simulink model "TestCurrentMotor"  (R2013b)
settings: Solver=ode45  StartTime=0.0  StopTime=inf  RelTol=1e-3
libraries: simulink x1
settings Model: Creator=eugenio  LastModifiedBy=eyime
settings DataIOCC: SignalLoggingSaveFormat=ModelDataLogs
settings OptimizationCC: ExpressionDepthLimit=2147483647
settings DebuggingCC: FcnCallInpInsideContextMsg=UseLocalSettings  StateNameClashWarn=warning
settings SFSimCC: SimParseCustomCode=off
settings GRTTargetCC: CombineOutputUpdateFcns=off  GRTInterface=on
settings SimMechanicsCC: VisDuringSimulation=on
settings ConfigurationSet: Description=SimMechanics 2G

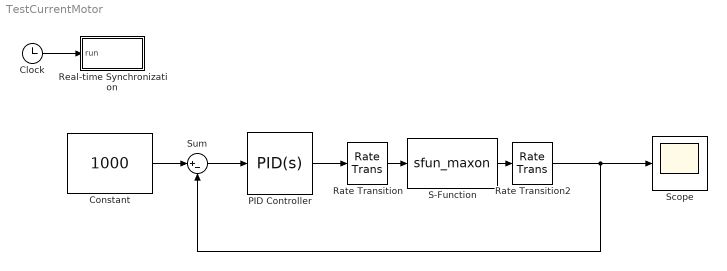
== system TestCurrentMotor ==
  Clock : Clock
  Constant : Constant  Value=1000
  PID Controller : simulink/Continuous/PID Controller  Controller=PID  TimeDomain=Continuous-time  SampleTime=1  IntegratorMethod=Forward Euler  FilterMethod=Forward Euler  Form=Parallel  P=0.1  I=0  D=0  N=100  InitialConditionSource=internal  InitialConditionForIntegrator=0  InitialConditionForFilter=0  ExternalReset=none  LimitOutput=off  UpperSaturationLimit=inf  LowerSaturationLimit=-inf  LinearizeAsGain=on  AntiWindupMode=none  Kb=1  TrackingMode=off  Kt=1  PParamMin=[]  PParamMax=[]  IParamMin=[]  IParamMax=[]  DParamMin=[]  DParamMax=[]  NParamMin=[]  NParamMax=[]  KbParamMin=[]  KbParamMax=[]  KtParamMin=[]  KtParamMax=[]  POutMin=[]  POutMax=[]  IOutMin=[]  IOutMax=[]  DOutMin=[]  DOutMax=[]  NOutMin=[]  NOutMax=[]  KbOutMin=[]  KbOutMax=[]  KtOutMin=[]  KtOutMax=[]  IntegratorOutMin=[]  IntegratorOutMax=[]  FilterOutMin=[]  FilterOutMax=[]  SumOutMin=[]  SumOutMax=[]  SumI1OutMin=[]  SumI1OutMax=[]  SumI2OutMin=[]  SumI2OutMax=[]  SumI3OutMin=[]  SumI3OutMax=[]  SumDOutMin=[]  SumDOutMax=[]  SaturationOutMin=[]  SaturationOutMax=[]  IntegratorContinuousStateAttributes=''  IntegratorStateMustResolveToSignalObject=off  IntegratorRTWStateStorageClass=Auto  FilterContinuousStateAttributes=''  FilterStateMustResolveToSignalObject=off  FilterRTWStateStorageClass=Auto
  Rate Transition : RateTransition
  Rate Transition2 : RateTransition
  Real-time Synchronization : Subsystem
  S-Function : S-Function  FunctionName=sfun_maxon  Parameters=NodeID, DeltaT, OpMode  EnableBusSupport=off  mask{NodeID=1, DeltaT=0.001, OpMode=1}
      mask prompts: DeltaT "Delta T"; OpMode "Operational Mode"
  Scope : Scope
      settings: YMin=3000  YMax=8000
  Sum : Sum  Inputs=|+-
  wires:
  Rate Transition/1 -> S-Function/1
  S-Function/1 -> Rate Transition2/1
  Rate Transition2/1 -> Sum/2, Scope/1
  Clock/1 -> Real-time Synchronization/1(run)
  Constant/1 -> Sum/1
  PID Controller/1 -> Rate Transition/1
  Sum/1 -> PID Controller/1

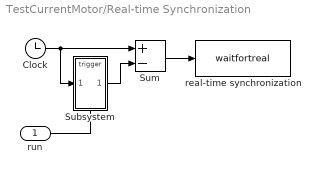
== system TestCurrentMotor/Real-time Synchronization ==
  run : Inport
  Clock : Clock
  Subsystem : Subsystem  TreatAsAtomicUnit=on
  Sum : Sum  Inputs=+-  SaturateOnIntegerOverflow=on  InputSameDT=on  OutDataTypeStr=Inherit: Same as first input
  real-time synchronization : MATLABFcn  MATLABFcn=waitfortreal  OutputDimensions=0
  wires:
  Clock/1 -> Subsystem/1(In), Sum/1
  Subsystem/1(Out) -> Sum/2
  Sum/1 -> real-time synchronization/1
  run/1 -> Subsystem/Trigger

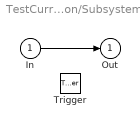
== system TestCurrentMotor/Real-time Synchronization/Subsystem ==
  In : Inport
  Trigger : TriggerPort
  Out : Outport  InitialOutput=0
  wires:
  In/1 -> Out/1
